simulink model "Model_LinearControl_Continous"  (R2019a)
settings: Solver=ode3  StartTime=0.0  StopTime=80  FixedStep=.001  RelTol=1e-3
undefined symbols (not defined in the file): Ap, Ar, At, Ax, Ay, Ayaw, Bp, Br, Bt, Bx, By, Byaw, CircleRadius, Ct, Cx, Cy, Dt, Dx, Dy, g, InputTransformation, InvT, Ixx, Iyy, Izz, Kp, Kr, Kt, Kx, Ky, Kyawc, Landingspeed, M, Mpayload, phi_init, phidot_init, psi_init, psidot_init, Squaremaxspeed, Squareminspeed, t_circle, t_landing, t_path, t_payloaddrop, t_squareLimit, t_takeoff, Takeoffspeed, theta_init, thetadot_init, TimePeriodCircle, x_init, xdot_init, y_init, ydot_init, z_init, zdot_init, zref_Landing, Zref_TakeOff
libraries: simulink x8
settings Model: Creator=c_satija  LastModifiedBy=Tasnim Haque
settings DataIOCC: SaveFormat=Array  SaveState=on
settings DebuggingCC: ArithmeticOperatorsInVariantConditions=warning
settings CodeAppCC: StateflowObjectComments=on

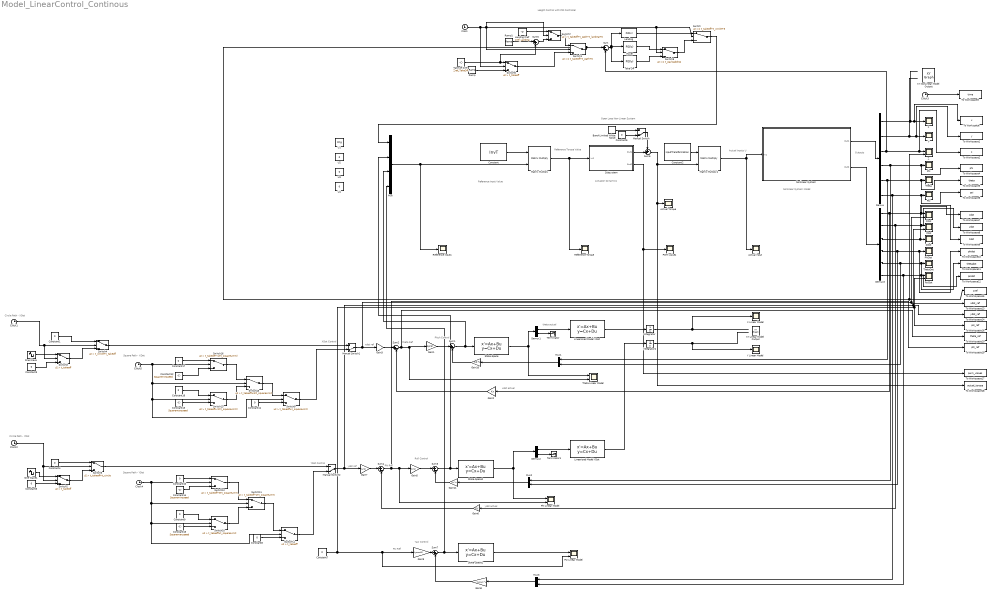
== system Model_LinearControl_Continous ==
  note: Square Path - YDot
  note: Square Path - XDot
  note: Circle Path - YDot
  note: Circle Path - XDot
  note: Psi Ref
  note: YDot Control
  note: XDot Control
  note: xdot ref
  note: xdot actual
  note: theta actual
  note: theta Ref
  note: Roll Control
  note: Pitch Control
  note: Open Loop Non-Linear System
  note: Height Control with PID Controller
  note: Actuator Dynamics
  note: Reference Input Value
  note: Reference
      | Torque Value
  note: Outputs
  note: Actual Inputs U
  note: Nonlinear System Model
  note: ydot actual
  note: ydot ref
  note: Phi Ref
  note: Yaw Control
  Actual Input : Scope
  Actual Torque : Scope
  Band-Limited White Noise : simulink/Sources/Band-Limited White Noise  Cov=[0.2]  Ts=.05  seed=[23341]
  Clock{,1..5} (6 alike) : Clock
  Constant : Constant  Value=InvT  VectorParams1D=off
  Constant{1,3..11,16..17} (12 alike) : Constant  Value=0
  Constant12 : Constant  Value=Squareminspeed
  Constant13 : Constant  Value=Squaremaxspeed
  Constant14 : Constant  Value=Squareminspeed
  Constant15 : Constant  Value=Squaremaxspeed
  Constant2 : Constant  Value=InputTransformation  VectorParams1D=off
  Demux : Demux  Outputs=6
  Demux1 : Demux  Outputs=2
  Demux2 : Demux  Outputs=2
  Demux3 : Demux  Outputs=6
  Gain1 : Gain  Gain=Kp(1)
  Gain10 : Gain  Gain=Kp  Multiplication=Matrix(K*u)
  Gain11 : Gain  Gain=Kr  Multiplication=Matrix(K*u)
  Gain2 : Gain  Gain=Kx
  Gain3 : Gain  Gain=Kx(1)
  Gain5 : Gain  Gain=Kr(1)
  Gain6 : Gain  Gain=Ky
  Gain7 : Gain  Gain=Ky(1)
  Gain8 : Gain  Gain=Kyawc  Multiplication=Matrix(K*u)
  Gain9 : Gain  Gain=Kyawc(1)
  Hover : simulink/Continuous/PID Controller  Controller=PID  Form=Parallel  TimeDomain=Continuous-time  SampleTime=-1  IntegratorMethod=Forward Euler  FilterMethod=Forward Euler  ControllerParametersSource=internal  P=60  I=10  D=20  UseFilter=on  N=1000  TunerSelectOption=Transfer Function Based (PID Tuner App)  ZeroCross=off  InitialConditionSource=internal  InitialConditionForIntegrator=0  InitialConditionForFilter=0  DifferentiatorICPrevScaledInput=0  ExternalReset=none  TrackingMode=off  Kt=1  LimitOutput=on  UpperSaturationLimit=24  LowerSaturationLimit=0  LinearizeAsGain=off  AntiWindupMode=none  Kb=1  POutMin=[]  POutMax=[]  IOutMin=[]  IOutMax=[]  DOutMin=[]  DOutMax=[]  NOutMin=[]  NOutMax=[]  SumOutMin=[]  SumOutMax=[]  SaturationOutMin=[]  SaturationOutMax=[]  PParamMin=[]  PParamMax=[]  IParamMin=[]  IParamMax=[]  DParamMin=[]  DParamMax=[]  NParamMin=[]  NParamMax=[]  KbParamMin=[]  KbParamMax=[]  KtParamMin=[]  KtParamMax=[]  KbOutMin=[]  KbOutMax=[]  KtOutMin=[]  KtOutMax=[]  IntegratorOutMin=[]  IntegratorOutMax=[]  FilterOutMin=[]  FilterOutMax=[]  SumI1OutMin=[]  SumI1OutMax=[]  SumI2OutMin=[]  SumI2OutMax=[]  SumI3OutMin=[]  SumI3OutMax=[]  SumI4OutMin=[]  SumI4OutMax=[]  SumDOutMin=[]  SumDOutMax=[]  DifferentiatorOutMin=[]  DifferentiatorOutMax=[]  FilterDiffOutCoefMin=[]  FilterDiffOutCoefMax=[]  ReciprocalOutMin=[]  ReciprocalOutMax=[]  SumDenOutMin=[]  SumDenOutMax=[]  SumNumOutMin=[]  SumNumOutMax=[]  DivideOutMin=[]  DivideOutMax=[]  IntegratorContinuousStateAttributes=''  IntegratorStateMustResolveToSignalObject=off  IntegratorRTWStateStorageClass=Auto  FilterContinuousStateAttributes=''  FilterStateMustResolveToSignalObject=off  FilterRTWStateStorageClass=Auto  ParallelPVariant=InternalParameters  IdealPVariant=Disabled  IVariant=InternalParameters  DVariant=InternalParameters  IntegratorVariant=Continuous  SatVariant=Enabled  AWVariant=Passthrough  PCopyVariant=Disabled  TRVariant=Disabled  FdbkBlocksVariant=Forward  IdealPFdbkVariant=Disabled  SatFdbkVariant=Disabled  DerivativeFilterVariant=ContFilter  NVariant=InternalParameters  NCopyVariant=Disabled  FilterICVariant=InternalICsFilter  IntegratorICVariant=InternalICs  ExternalResetVariant=Disabled  TRSumVariant=Passthrough  SumFdbkVariant=Disabled  SumVariant=Sum_PID
  Integrator : Integrator  InitialCondition=x_init
  Integrator2 : Integrator  InitialCondition=y_init
  Landing : simulink/Continuous/PID Controller  Controller=PID  Form=Parallel  TimeDomain=Continuous-time  SampleTime=-1  IntegratorMethod=Forward Euler  FilterMethod=Forward Euler  ControllerParametersSource=internal  P=60  I=10  D=25  UseFilter=on  N=1000  TunerSelectOption=Transfer Function Based (PID Tuner App)  ZeroCross=off  InitialConditionSource=internal  InitialConditionForIntegrator=0  InitialConditionForFilter=0  DifferentiatorICPrevScaledInput=0  ExternalReset=none  TrackingMode=off  Kt=1  LimitOutput=on  UpperSaturationLimit=24  LowerSaturationLimit=0  LinearizeAsGain=off  AntiWindupMode=none  Kb=1  POutMin=[]  POutMax=[]  IOutMin=[]  IOutMax=[]  DOutMin=[]  DOutMax=[]  NOutMin=[]  NOutMax=[]  SumOutMin=[]  SumOutMax=[]  SaturationOutMin=[]  SaturationOutMax=[]  PParamMin=[]  PParamMax=[]  IParamMin=[]  IParamMax=[]  DParamMin=[]  DParamMax=[]  NParamMin=[]  NParamMax=[]  KbParamMin=[]  KbParamMax=[]  KtParamMin=[]  KtParamMax=[]  KbOutMin=[]  KbOutMax=[]  KtOutMin=[]  KtOutMax=[]  IntegratorOutMin=[]  IntegratorOutMax=[]  FilterOutMin=[]  FilterOutMax=[]  SumI1OutMin=[]  SumI1OutMax=[]  SumI2OutMin=[]  SumI2OutMax=[]  SumI3OutMin=[]  SumI3OutMax=[]  SumI4OutMin=[]  SumI4OutMax=[]  SumDOutMin=[]  SumDOutMax=[]  DifferentiatorOutMin=[]  DifferentiatorOutMax=[]  FilterDiffOutCoefMin=[]  FilterDiffOutCoefMax=[]  ReciprocalOutMin=[]  ReciprocalOutMax=[]  SumDenOutMin=[]  SumDenOutMax=[]  SumNumOutMin=[]  SumNumOutMax=[]  DivideOutMin=[]  DivideOutMax=[]  IntegratorContinuousStateAttributes=''  IntegratorStateMustResolveToSignalObject=off  IntegratorRTWStateStorageClass=Auto  FilterContinuousStateAttributes=''  FilterStateMustResolveToSignalObject=off  FilterRTWStateStorageClass=Auto  ParallelPVariant=InternalParameters  IdealPVariant=Disabled  IVariant=InternalParameters  DVariant=InternalParameters  IntegratorVariant=Continuous  SatVariant=Enabled  AWVariant=Passthrough  PCopyVariant=Disabled  TRVariant=Disabled  FdbkBlocksVariant=Forward  IdealPFdbkVariant=Disabled  SatFdbkVariant=Disabled  DerivativeFilterVariant=ContFilter  NVariant=InternalParameters  NCopyVariant=Disabled  FilterICVariant=InternalICsFilter  IntegratorICVariant=InternalICs  ExternalResetVariant=Disabled  TRSumVariant=Passthrough  SumFdbkVariant=Disabled  SumVariant=Sum_PID
  Landing Zref : Constant  Value=zref_Landing
  Linearised Model YDot : StateSpace  A=Ay  B=By  C=Cy  D=Dy  InitialCondition=[xdot_init]
  Linearozed Model XDot : StateSpace  A=Ax  B=Bx  C=Cx  D=Dx  InitialCondition=[xdot_init]
  Manual Switch : ManualSwitch  CurrentSetting=0
  Manual Switch1 : ManualSwitch  CurrentSetting=0
  Manual Switch2 : ManualSwitch  CurrentSetting=0
  Matrix Multiply : Product  Multiplication=Matrix(*)
  Matrix Multiply1 : Product  Multiplication=Matrix(*)
  Mux : Mux
  Mux1 : Mux  Inputs=2
  Mux2 : Mux  Inputs=2
  Mux3 : Mux  Inputs=2
  Nonlinear System : Subsystem
  PWM values : Scope
  Phi : Scope
  Phi Linear Model : Scope  NumInputPorts=2
  PhiDot : Scope
  Psi : Scope
  Psi Linear Model : Scope  NumInputPorts=2
  PsiDot : Scope  NumInputPorts=2
  Ramp : simulink/Sources/Ramp  slope=Takeoffspeed  start=0  InitialOutput=0
  Ramp1 : simulink/Sources/Ramp  slope=Landingspeed  start=t_takeoff+t_path+5  InitialOutput=0
  Reference Inputs : Scope
  Reference Torque : Scope
  Sine Wave : Sin  Amplitude=((2*pi)/TimePeriodCircle)*CircleRadius  Frequency=(2*pi)/TimePeriodCircle  SampleTime=0
  Sine Wave1 : Sin  Amplitude=((2*pi)/TimePeriodCircle)*CircleRadius  Frequency=(2*pi)/TimePeriodCircle  Phase=pi/2  SampleTime=0
  State-Space : StateSpace  A=Ap  B=Bp  C=eye(2)  D=[0;0]  InitialCondition=[theta_init;thetadot_init]
  State-Space1 : StateSpace  A=Ayaw  B=Byaw  C=eye(2)  D=[0;0]  InitialCondition=[psi_init;psidot_init]
  State-Space2 : StateSpace  A=Ar  B=Br  C=eye(2)  D=[0;0]  InitialCondition=[phi_init;phidot_init]
  Subsystem : Subsystem
  Sum{,1..4,7} (6 alike) : Sum  Inputs=|+-
  Sum5 : Sum  Inputs=|++
  Sum6 : Sum  Inputs=++|
  Switch : Switch  Threshold=t_takeoff+t_circle+5
  Switch1 : Switch  Threshold=t_takeoff+t_path+5
  Switch10 : Switch  Criteria=u2 > Threshold  Threshold=t_takeoff+t_squareLimit
  Switch11 : Switch  Criteria=u2 > Threshold  Threshold=t_takeoff+2*t_squareLimit
  Switch12 : Switch  Criteria=u2 > Threshold  Threshold=t_takeoff+3*t_squareLimit
  Switch13 : Switch  Criteria=u2 > Threshold  Threshold=t_takeoff+(2*t_squareLimit)
  Switch{2..3,6,14} (4 alike) : Switch  Criteria=u2 > Threshold  Threshold=t_takeoff
  Switch15 : Switch  Criteria=u2 > Threshold  Threshold=t_takeoff+3*t_squareLimit
  Switch16 : Switch  Criteria=u2 > Threshold  Threshold=t_takeoff+(4*t_squareLimit)
  Switch4 : Switch  Criteria=u2 > Threshold  Threshold=t_circle+t_takeoff
  Switch5 : Switch  Criteria=u2 > Threshold  Threshold=t_takeoff+t_circle
  Switch7 : Switch  Criteria=u2 > Threshold  Threshold=t_takeoff+t_path+t_landing+5
  Switch8 : Switch  Threshold=t_payloaddrop
  Switch9 : Switch  Criteria=u2 > Threshold  Threshold=t_takeoff+t_squareLimit
  "Take Off " : simulink/Continuous/PID Controller  Controller=PID  Form=Parallel  TimeDomain=Continuous-time  SampleTime=-1  IntegratorMethod=Forward Euler  FilterMethod=Forward Euler  ControllerParametersSource=internal  P=60  I=10  D=20  UseFilter=on  N=1000  TunerSelectOption=Transfer Function Based (PID Tuner App)  ZeroCross=off  InitialConditionSource=internal  InitialConditionForIntegrator=0  InitialConditionForFilter=0  DifferentiatorICPrevScaledInput=0  ExternalReset=none  TrackingMode=off  Kt=1  LimitOutput=on  UpperSaturationLimit=24  LowerSaturationLimit=0  LinearizeAsGain=off  AntiWindupMode=none  Kb=1  POutMin=[]  POutMax=[]  IOutMin=[]  IOutMax=[]  DOutMin=[]  DOutMax=[]  NOutMin=[]  NOutMax=[]  SumOutMin=[]  SumOutMax=[]  SaturationOutMin=[]  SaturationOutMax=[]  PParamMin=[]  PParamMax=[]  IParamMin=[]  IParamMax=[]  DParamMin=[]  DParamMax=[]  NParamMin=[]  NParamMax=[]  KbParamMin=[]  KbParamMax=[]  KtParamMin=[]  KtParamMax=[]  KbOutMin=[]  KbOutMax=[]  KtOutMin=[]  KtOutMax=[]  IntegratorOutMin=[]  IntegratorOutMax=[]  FilterOutMin=[]  FilterOutMax=[]  SumI1OutMin=[]  SumI1OutMax=[]  SumI2OutMin=[]  SumI2OutMax=[]  SumI3OutMin=[]  SumI3OutMax=[]  SumI4OutMin=[]  SumI4OutMax=[]  SumDOutMin=[]  SumDOutMax=[]  DifferentiatorOutMin=[]  DifferentiatorOutMax=[]  FilterDiffOutCoefMin=[]  FilterDiffOutCoefMax=[]  ReciprocalOutMin=[]  ReciprocalOutMax=[]  SumDenOutMin=[]  SumDenOutMax=[]  SumNumOutMin=[]  SumNumOutMax=[]  DivideOutMin=[]  DivideOutMax=[]  IntegratorContinuousStateAttributes=''  IntegratorStateMustResolveToSignalObject=off  IntegratorRTWStateStorageClass=Auto  FilterContinuousStateAttributes=''  FilterStateMustResolveToSignalObject=off  FilterRTWStateStorageClass=Auto  ParallelPVariant=InternalParameters  IdealPVariant=Disabled  IVariant=InternalParameters  DVariant=InternalParameters  IntegratorVariant=Continuous  SatVariant=Enabled  AWVariant=Passthrough  PCopyVariant=Disabled  TRVariant=Disabled  FdbkBlocksVariant=Forward  IdealPFdbkVariant=Disabled  SatFdbkVariant=Disabled  DerivativeFilterVariant=ContFilter  NVariant=InternalParameters  NCopyVariant=Disabled  FilterICVariant=InternalICsFilter  IntegratorICVariant=InternalICs  ExternalResetVariant=Disabled  TRSumVariant=Passthrough  SumFdbkVariant=Disabled  SumVariant=Sum_PID
  Take off Zref : Constant  Value=Zref_TakeOff
  Terminator : Terminator
  Terminator1 : Terminator
  Theta : Scope
  "Theta Linear Model " : Scope  NumInputPorts=2
  ThetaDot : Scope
  To Workspace : ToWorkspace  VariableName=x  SampleTime=-1
  To Workspace1 : ToWorkspace  VariableName=y  SampleTime=-1
  To Workspace10 : ToWorkspace  VariableName=phidot  SampleTime=-1
  To Workspace11 : ToWorkspace  VariableName=thetadot  SampleTime=-1
  To Workspace12 : ToWorkspace  VariableName=psidot  SampleTime=-1
  To Workspace13 : ToWorkspace  VariableName=xdot_ref  SampleTime=-1
  To Workspace14 : ToWorkspace  VariableName=ydot_ref  SampleTime=-1
  To Workspace15 : ToWorkspace  VariableName=zref  SampleTime=-1
  To Workspace16 : ToWorkspace  VariableName=psi_ref  SampleTime=-1
  To Workspace17 : ToWorkspace  VariableName=pwm_values  SampleTime=-1
  To Workspace18 : ToWorkspace  VariableName=actual_torque  SampleTime=-1
  To Workspace19 : ToWorkspace  VariableName=phi_ref  SampleTime=-1
  To Workspace2 : ToWorkspace  VariableName=z  SampleTime=-1
  To Workspace20 : ToWorkspace  VariableName=theta_ref  SampleTime=-1
  To Workspace3 : ToWorkspace  VariableName=time  SaveFormat=Timeseries  SampleTime=-1
  To Workspace4 : ToWorkspace  VariableName=phi  SampleTime=-1
  To Workspace5 : ToWorkspace  VariableName=theta  SampleTime=-1
  To Workspace6 : ToWorkspace  VariableName=psi  SampleTime=-1
  To Workspace7 : ToWorkspace  VariableName=xdot  SampleTime=-1
  To Workspace8 : ToWorkspace  VariableName=ydot  SampleTime=-1
  To Workspace9 : ToWorkspace  VariableName=zdot  SampleTime=-1
  U1 : Constant  Value=M*g
  U2 : Constant  Value=0
  U3 : Constant  Value=0
  U4 : Constant  Value=0
  X : Scope
  X Linear Model : Scope
  XDot : Scope  NumInputPorts=2
  XY Linear Model Output : simulink/Sinks/XY Graph  xmin=-10  xmax=10  ymin=-10  ymax=10  st=-1
  XY NonLinear Model Output : simulink/Sinks/XY Graph  xmin=-5  xmax=5  ymin=-5  ymax=5  st=-1
  Y : Scope
  Y Linear Model : Scope
  YDot : Scope  NumInputPorts=2
  Z : Scope  NumInputPorts=2
  ZDot : Scope
  wires:
  Constant/1 -> Matrix Multiply/1
  Matrix Multiply/1 -> Reference Torque/1, Subsystem/1(In2)
  Demux/5 -> Mux1/1, To Workspace5/1, Theta/1
  Demux/6 -> To Workspace6/1, Psi/1, Mux3/1
  Sum/1 -> Hover/1, Landing/1, "Take Off "/1
  Clock/1 -> Switch1/2, Switch7/2, Switch8/2, Switch/2, Switch6/2
  Switch/1 -> Mux/1
  Switch1/1 -> Sum/1, Z/2, To Workspace15/1
  Demux/4 -> Mux2/1, To Workspace4/1, Phi/1
  Demux/3 -> To Workspace2/1, Z/1, Sum/2
  Demux/2 -> Y/1, To Workspace1/1
  Demux/1 -> X/1, To Workspace/1
  Mux/1 -> Reference Inputs/1, Matrix Multiply/2
  Nonlinear System/1(Out1) -> Demux/1
  Constant2/1 -> Matrix Multiply1/1
  Matrix Multiply1/1 -> Nonlinear System/1(In1), Actual Input/1
  Subsystem/2(Out2) -> PWM values/1, To Workspace17/1
  Landing/1 -> Switch/1
  State-Space/1 -> "Theta Linear Model "/1, Demux1/1
  Sum1/1 -> Mux/3, State-Space/1
  Sum2/1 -> To Workspace20/1, Gain1/1, "Theta Linear Model "/2
  Gain1/1 -> Sum1/1
  Demux1/2 -> Terminator/1
  Demux1/1 -> Linearozed Model XDot/1
  Linearozed Model XDot/1 -> Integrator/1
  Sine Wave/1 -> Switch3/1
  Gain2/1 -> Sum2/2
  Gain3/1 -> Sum2/1
  Demux2/2 -> Terminator1/1
  Manual Switch2/1 -> Gain7/1, To Workspace14/1, YDot/2
  Linearised Model YDot/1 -> Integrator2/1
  Demux2/1 -> Linearised Model YDot/1
  Gain6/1 -> Sum4/2
  Gain5/1 -> Sum3/1
  Gain7/1 -> Sum4/1
  Sum3/1 -> State-Space2/1, Mux/2
  State-Space2/1 -> Demux2/1, Phi Linear Model/1
  Sum4/1 -> To Workspace19/1, Phi Linear Model/2, Gain5/1
  Integrator/1 -> X Linear Model/1
  Integrator2/1 -> Y Linear Model/1
  Nonlinear System/2(Out2) -> Demux3/1
  Demux3/1 -> To Workspace7/1, XDot/1, Gain2/1
  Demux3/2 -> Gain6/1, To Workspace8/1, YDot/1
  Manual Switch1/1 -> Gain3/1, XDot/2, To Workspace13/1
  Clock1/1 -> Switch4/2, Switch3/2
  Constant3/1 -> Switch3/3
  Constant1/1 -> Switch4/1
  Switch3/1 -> Switch4/3
  Constant5/1 -> Switch2/3
  Clock2/1 -> Switch2/2, Switch5/2
  Sine Wave1/1 -> Switch2/1
  Constant4/1 -> Switch5/1
  Switch2/1 -> Switch5/3
  Clock3/1 -> To Workspace3/1
  Ramp/1 -> Switch6/3
  Take off Zref/1 -> Sum5/2, Switch6/1
  Switch6/1 -> Switch1/3
  Landing Zref/1 -> Switch7/1
  Switch7/1 -> Switch1/1
  Demux3/3 -> ZDot/1, To Workspace9/1
  Ramp1/1 -> Sum5/1
  Sum5/1 -> Switch7/3
  Demux3/4 -> Mux2/2, PhiDot/1, To Workspace10/1
  Demux3/5 -> ThetaDot/1, To Workspace11/1, Mux1/2
  Demux3/6 -> To Workspace12/1, PsiDot/1, Mux3/2
  Subsystem/1(Out1) -> Sum6/2
  Sum6/1 -> Matrix Multiply1/2, Actual Torque/1, To Workspace18/1
  Band-Limited White Noise/1 -> Manual Switch/1
  Manual Switch/1 -> Sum6/1
  Constant6/1 -> Manual Switch/2
  Gain8/1 -> Sum7/2
  Gain9/1 -> Sum7/1
  State-Space1/1 -> Psi Linear Model/1
  Switch8/1 -> Switch/3
  "Take Off "/1 -> Switch8/3
  Hover/1 -> Switch8/1
  Sum7/1 -> State-Space1/1, Mux/4
  Constant7/1 -> To Workspace16/1, PsiDot/2, Gain9/1, Psi Linear Model/2
  Gain11/1 -> Sum3/2
  Gain10/1 -> Sum1/2
  Mux1/1 -> Gain10/1
  Mux2/1 -> Gain11/1
  Mux3/1 -> Gain8/1
  Switch4/1 -> Manual Switch1/1
  Switch5/1 -> Manual Switch2/1
  Constant8/1 -> Switch14/3
  Clock4/1 -> Switch14/2, Switch10/2, Switch11/2, Switch12/2
  Constant9/1 -> Switch10/1
  Switch10/1 -> Switch11/3
  Switch11/1 -> Switch14/1
  Constant10/1 -> Switch12/1
  Constant11/1 -> Switch9/3
  Clock5/1 -> Switch13/2, Switch9/2, Switch15/2, Switch16/2
  Constant16/1 -> Switch13/1
  Switch13/1 -> Switch15/3
  Switch15/1 -> Switch9/1
  Constant17/1 -> Switch16/1
  Switch14/1 -> Manual Switch2/2
  Switch9/1 -> Manual Switch1/2
  Switch16/1 -> Switch15/1
  Switch12/1 -> Switch11/1
  Constant12/1 -> Switch16/3
  Constant13/1 -> Switch13/3
  Constant14/1 -> Switch12/3
  Constant15/1 -> Switch10/3

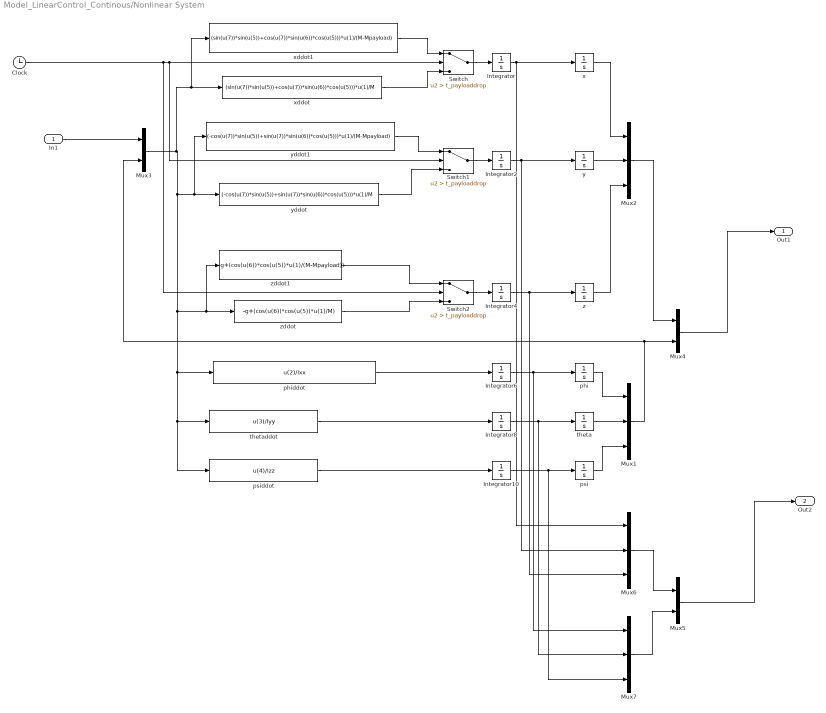
== system Model_LinearControl_Continous/Nonlinear System ==
  In1 : Inport
  Clock : Clock
  Integrator : Integrator  InitialCondition=xdot_init
  Integrator10 : Integrator  InitialCondition=psidot_init
  Integrator2 : Integrator  InitialCondition=ydot_init
  Integrator4 : Integrator  InitialCondition=zdot_init
  Integrator6 : Integrator  InitialCondition=phidot_init
  Integrator8 : Integrator  InitialCondition=thetadot_init
  Mux{1..2,6..7} (4 alike) : Mux  Inputs=3
  Mux3 : Mux  Inputs=2
  Mux4 : Mux  Inputs=2
  Mux5 : Mux  Inputs=2
  Switch : Switch  Criteria=u2 > Threshold  Threshold=t_payloaddrop
  Switch1 : Switch  Criteria=u2 > Threshold  Threshold=t_payloaddrop
  Switch2 : Switch  Criteria=u2 > Threshold  Threshold=t_payloaddrop
  phi : Integrator  InitialCondition=phi_init
  phiddot : Fcn  Expr=u(2)/Ixx
  psi : Integrator  InitialCondition=psi_init
  psiddot : Fcn  Expr=u(4)/Izz
  theta : Integrator  InitialCondition=theta_init
  thetaddot : Fcn  Expr=u(3)/Iyy
  x : Integrator  InitialCondition=x_init
  xddot : Fcn  Expr=(sin(u(7))*sin(u(5))+cos(u(7))*sin(u(6))*cos(u(5)))*u(1)/M
  xddot1 : Fcn  Expr=(sin(u(7))*sin(u(5))+cos(u(7))*sin(u(6))*cos(u(5)))*u(1)/(M-Mpayload)
  y : Integrator  InitialCondition=y_init
  yddot : Fcn  Expr=(-cos(u(7))*sin(u(5))+sin(u(7))*sin(u(6))*cos(u(5)))*u(1)/M
  yddot1 : Fcn  Expr=(-cos(u(7))*sin(u(5))+sin(u(7))*sin(u(6))*cos(u(5)))*u(1)/(M-Mpayload)
  z : Integrator  InitialCondition=z_init
  zddot : Fcn  Expr=-g+(cos(u(6))*cos(u(5))*u(1)/M)
  zddot1 : Fcn  Expr=-g+(cos(u(6))*cos(u(5))*u(1)/(M-Mpayload))
  Out1 : Outport
  Out2 : Outport  Port=2
  wires:
  Mux1/1 -> Mux4/2, Mux3/2
  Mux4/1 -> Out1/1
  Mux3/1 -> yddot1/1, yddot/1, zddot1/1, zddot/1, phiddot/1, thetaddot/1, psiddot/1, xddot/1, xddot1/1
  x/1 -> Mux2/1
  zddot/1 -> Switch2/3
  Integrator/1 -> Mux6/1, x/1
  Integrator2/1 -> y/1, Mux6/2
  Mux2/1 -> Mux4/1
  phi/1 -> Mux1/1
  psiddot/1 -> Integrator10/1
  thetaddot/1 -> Integrator8/1
  Integrator6/1 -> phi/1, Mux7/1
  psi/1 -> Mux1/3
  Integrator8/1 -> theta/1, Mux7/2
  theta/1 -> Mux1/2
  y/1 -> Mux2/2
  phiddot/1 -> Integrator6/1
  Integrator10/1 -> psi/1, Mux7/3
  Integrator4/1 -> Mux6/3, z/1
  yddot/1 -> Switch1/3
  z/1 -> Mux2/3
  In1/1 -> Mux3/1
  Mux6/1 -> Mux5/1
  Mux7/1 -> Mux5/2
  Mux5/1 -> Out2/1
  Switch/1 -> Integrator/1
  xddot/1 -> Switch/3
  Switch1/1 -> Integrator2/1
  Switch2/1 -> Integrator4/1
  yddot1/1 -> Switch1/1
  xddot1/1 -> Switch/1
  zddot1/1 -> Switch2/1
  Clock/1 -> Switch/2, Switch1/2, Switch2/2

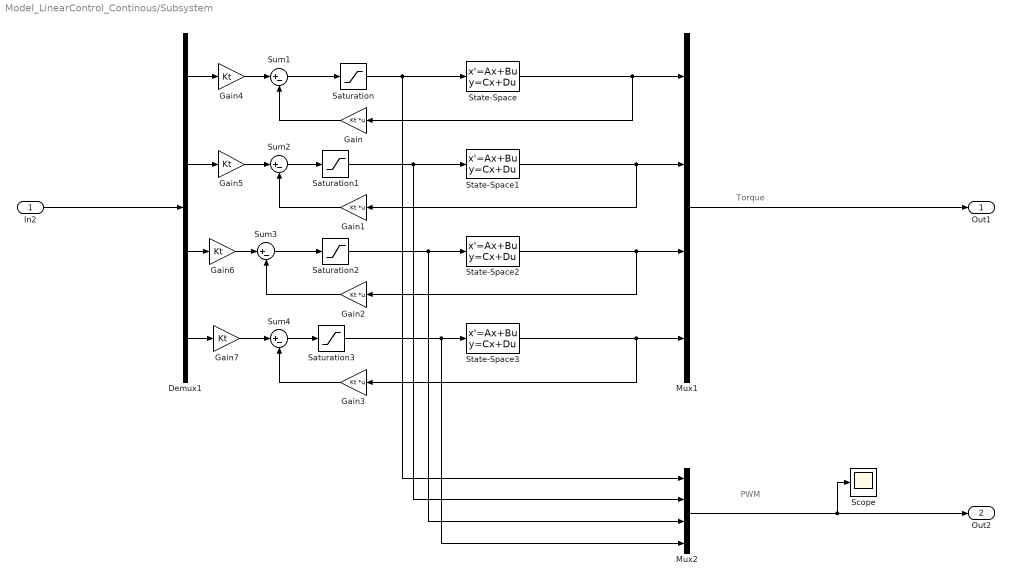
== system Model_LinearControl_Continous/Subsystem ==
  note: PWM
  note: Torque
  In2 : Inport
  Demux1 : Demux
  Gain{,1..3} (4 alike) : Gain  Gain=Kt  Multiplication=Matrix(K*u)
  Gain{4..7} (4 alike) : Gain  Gain=Kt
  Mux1 : Mux
  Mux2 : Mux
  Saturation{,1..3} (4 alike) : Saturate  UpperLimit=0.05  LowerLimit=0  LinearizeAsGain=off  ZeroCross=off  OutMin=[0]  OutMax=[0.05]
  Scope : Scope
  State-Space{,1..3} (4 alike) : StateSpace  A=At  B=Bt  C=Ct  D=Dt  InitialCondition=0
  Sum{1..4} (4 alike) : Sum  Inputs=|+-
  Out1 : Outport
  Out2 : Outport  Port=2
  wires:
  In2/1 -> Demux1/1
  Demux1/1 -> Gain4/1
  Mux1/1 -> Out1/1
  Sum1/1 -> Saturation/1
  State-Space/1 -> Gain/1, Mux1/1
  State-Space1/1 -> Mux1/2, Gain1/1
  Demux1/2 -> Gain5/1
  Sum2/1 -> Saturation1/1
  State-Space2/1 -> Mux1/3, Gain2/1
  Demux1/3 -> Gain6/1
  Sum3/1 -> Saturation2/1
  State-Space3/1 -> Mux1/4, Gain3/1
  Demux1/4 -> Gain7/1
  Sum4/1 -> Saturation3/1
  Mux2/1 -> Scope/1, Out2/1
  Gain/1 -> Sum1/2
  Gain1/1 -> Sum2/2
  Gain2/1 -> Sum3/2
  Gain3/1 -> Sum4/2
  Gain4/1 -> Sum1/1
  Gain5/1 -> Sum2/1
  Gain6/1 -> Sum3/1
  Gain7/1 -> Sum4/1
  Saturation/1 -> State-Space/1, Mux2/1
  Saturation1/1 -> State-Space1/1, Mux2/2
  Saturation2/1 -> State-Space2/1, Mux2/3
  Saturation3/1 -> State-Space3/1, Mux2/4
